simulink model "CF010A_GmTqArbn"  (R2013b)
settings: Solver=FixedStepDiscrete  SolverMode=SingleTasking  StartTime=0.0  StopTime=1  FixedStep=0.002  RelTol=1e-3
values from neighbouring files (symbols this model uses):
  ARCHGLBPRM_2MILLISEC_SEC_F32 = DataDict.Constant    [CF010A_GmTqArbn_DataDict.m]
  ESCCMDACTV_CNT_U08 = DataDict.Constant    [CF010A_GmTqArbn_DataDict.m]
  ESCCMDTMPLIMD_CNT_U08 = DataDict.Constant    [CF010A_GmTqArbn_DataDict.m]
  ESCTQCMDOVRLLIM_HWNWTMTR_F32 = DataDict.Constant    [CF010A_GmTqArbn_DataDict.m]
  FINALSLEWLWRLIM_HWNWTMTRPERSEC_F32 = DataDict.Constant    [CF010A_GmTqArbn_DataDict.m]
  GmTqArbnApaAssiScaEna = DataDict.Calibration    [CF010A_GmTqArbn_DataDict.m]
  GmTqArbnApaDampgScaEna = DataDict.Calibration    [CF010A_GmTqArbn_DataDict.m]
  GmTqArbnApaEnaRate = DataDict.Calibration    [CF010A_GmTqArbn_DataDict.m]
  GmTqArbnApaRtnScaEna = DataDict.Calibration    [CF010A_GmTqArbn_DataDict.m]
  GmTqArbnEscMaxTq = DataDict.Calibration    [CF010A_GmTqArbn_DataDict.m]
  GmTqArbnLkaSlewEna = DataDict.Calibration    [CF010A_GmTqArbn_DataDict.m]
  HWTQCMDOVRLLIM_HWNWTMTR_F32 = DataDict.Constant    [CF010A_GmTqArbn_DataDict.m]
  LKACMDHILIM_HWNWTMTR_F32 = DataDict.Constant    [CF010A_GmTqArbn_DataDict.m]
  LKASTACTV_CNT_U08 = DataDict.Constant    [CF010A_GmTqArbn_DataDict.m]
  LKATQCMDOVRLLIM_HWNWTMTR_F32 = DataDict.Constant    [CF010A_GmTqArbn_DataDict.m]
  MOTTQCMDOVRLLIM_MOTNWTMTR_F32 = DataDict.Constant    [CF010A_GmTqArbn_DataDict.m]
  OUTPCMDHILIM_ULS_F32 = DataDict.Constant    [CF010A_GmTqArbn_DataDict.m]
  OUTPCMDLOWRLIM_ULS_F32 = DataDict.Constant    [CF010A_GmTqArbn_DataDict.m]
  POSNSERVOSMOOTHMINLWRLIM_ULSPERSEC_F32 = DataDict.Constant    [CF010A_GmTqArbn_DataDict.m]
  VELDPTTQOVRLMTRCOFFS_HWNWTMTRPERSEC_F32 = DataDict.Constant    [CF010A_GmTqArbn_DataDict.m]
  VELDPTTQOVRLMTRCTQPERVEHSPD_HWNWTMTRPERSECPERKPH_F32 = DataDict.Constant    [CF010A_GmTqArbn_DataDict.m]
libraries: NxtrLim x11, NexteerUtilities x8, FixdToFloat x3, Fil x2, NxtrAbslt x2, simulink x2
(part 2 of 4)

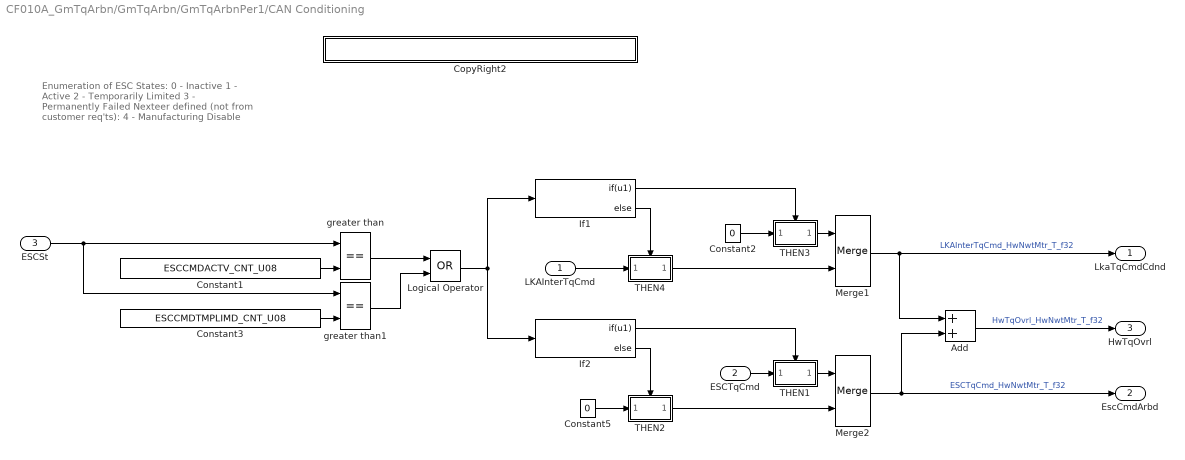
== system CF010A_GmTqArbn/GmTqArbn/GmTqArbnPer1/CAN Conditioning ==
  note: Enumeration of ESC States:
      |     0 - Inactive
      |     1 - Active
      |     2 - Temporarily Limited
      |     3 - Permanently Failed
      |
      | Nexteer defined (not from customer req'ts):
      |     4 - Manufacturing Disable
  LKAInterTqCmd : Inport
  ESCTqCmd : Inport  Port=2
  ESCSt : Inport  Port=3
  Add : Sum
  Constant1 : Constant  Value=ESCCMDACTV_CNT_U08
  Constant2 : Constant  Value=0  OutDataTypeStr=single
  Constant3 : Constant  Value=ESCCMDTMPLIMD_CNT_U08
  Constant5 : Constant  Value=0  OutDataTypeStr=single
  CopyRight2 : Subsystem  Description=|  mask(Copyright Information){none=on}
      | Copyright info block.                                               
      |                                                                     
      | Place copyright information at the top of every subsystem in design.
      mask prompts: none "No parameters"
      mask help: Place copyright information at the top of every subsystem in design.
      mask Display:
      | NxtrConf = 'Nexteer Confidential';
      | 
      | sys = bdroot; %handle for the current model ("system")
      | first = get_param(sys,'Created');
      | first = first(end-3:end);  %year is last four digits
      | 
      | last = get_param(sys,'LastModifiedDate');
      | if isempty(last)
      |     last = datestr(now,'yyyy');
      | else
      |     last = last(end-3:end);
      | end
      | 
      | if strcmp(first,last)
      |     fprintf('%s -- Copyright %s Nexteer',NxtrConf,first)
      | else
      |     fprintf('%s -- %s%s- %s Nexteer',NxtrConf,char(169),first,last)
      | end
  If1 : If  IfExpression=u1
  If2 : If  IfExpression=u1
  Logical Operator : Logic  Operator=OR  AllPortsSameDT=off  OutDataTypeStr=boolean
  Merge1 : Merge
  Merge2 : Merge
  THEN1 : Subsystem  RequirementInfo={} %GIDa_df789066_5626_4b2f_a61b_8784029d3cc8  TreatAsAtomicUnit=on  mask(pass thru, version Nov 30, 2012){nIn=1}
      mask prompts: nIn "Number of input signals"
      mask help:
      | This block passes its input straight through without modification.
      |
      | Enter the number of signals to pass through (integer 1 to 5).
      mask Callback nIn:
      | thisBlock = gcb;
      | a = get_param(thisBlock,'MaskValues');
      | b = cell2mat(a);
      | c = str2num(b);
      | 
      | if c<1 c=1; end
      | if c>5 c=5; end
      | 
      | for idx=1:c
      |     sIdx = num2str(idx);
      |     oldblock = [thisBlock '/In' sIdx];
      |     if strcmp(get_param(oldblock,'BlockType'),'Ground')
      |          newblock = 'built-in/Inport';
      |         pos = get_param(oldblock,'Position');
      |         orient = get_param(oldblock,'Orientation');
      |         delete_block(oldblock);
      |         add_block(newblock,oldblock,'Position',pos, 'Orientation',orient);
      |     end
      | 
      |     oldblock = [thisBlock '/Out' sIdx];
      |     if strcmp(get_param(oldblock,'BlockType'),'Terminator')
      |         newblock = 'built-in/Outport';
      |         pos = get_param(oldblock,'Position');
      |         orient = get_param(oldblock,'Orientation');
      |         delete_block(oldblock);
      |         add_block(newblock,oldblock,'Position',pos, 'Orientation',orient);
      |     end
      | end
      | 
      | for idx=c+1:5
      |     sIdx = num2str(idx);
      |     oldblock = [thisBlock '/In' sIdx];
      |     if strcmp(get_param(oldblock,'BlockType'),'Inport')
      |         newblock = 'built-in/Ground';
      |         pos = get_param(oldblock,'Position');
      |         orient = get_param(oldblock,'Orientation');
      |         delete_block(oldblock);
      |         add_block(newblock,oldblock,'Position',pos, 'Orientation',orient);
      |     end
      | 
      |     oldblock = [thisBlock '/Out' sIdx];
      |     if strcmp(get_param(oldblock,'BlockType'),'Outport')
      |         newblock = 'built-in/Terminator';
      |         pos = get_param(oldblock,'Position');
      |         orient = get_param(oldblock,'Orientation');
      |         delete_block(oldblock);
      |         add_block(newblock,oldblock,'Position',pos, 'Orientation',orient);
      |     end
      | end
      | 
      | 
      | 
      | clear thisBlock oldblock newblock orient pos a b c idx sIdx ;
      mask Display: fprintf('pass\nthru')
  THEN2 : Subsystem  RequirementInfo={} %GIDa_50ca75fe_c393_440b_9fca_2138a66effba  TreatAsAtomicUnit=on  mask(pass thru, version Nov 30, 2012){nIn=1}
      mask prompts: nIn "Number of input signals"
      mask help:
      | This block passes its input straight through without modification.
      |
      | Enter the number of signals to pass through (integer 1 to 5).
      mask Callback nIn:
      | thisBlock = gcb;
      | a = get_param(thisBlock,'MaskValues');
      | b = cell2mat(a);
      | c = str2num(b);
      | 
      | if c<1 c=1; end
      | if c>5 c=5; end
      | 
      | for idx=1:c
      |     sIdx = num2str(idx);
      |     oldblock = [thisBlock '/In' sIdx];
      |     if strcmp(get_param(oldblock,'BlockType'),'Ground')
      |          newblock = 'built-in/Inport';
      |         pos = get_param(oldblock,'Position');
      |         orient = get_param(oldblock,'Orientation');
      |         delete_block(oldblock);
      |         add_block(newblock,oldblock,'Position',pos, 'Orientation',orient);
      |     end
      | 
      |     oldblock = [thisBlock '/Out' sIdx];
      |     if strcmp(get_param(oldblock,'BlockType'),'Terminator')
      |         newblock = 'built-in/Outport';
      |         pos = get_param(oldblock,'Position');
      |         orient = get_param(oldblock,'Orientation');
      |         delete_block(oldblock);
      |         add_block(newblock,oldblock,'Position',pos, 'Orientation',orient);
      |     end
      | end
      | 
      | for idx=c+1:5
      |     sIdx = num2str(idx);
      |     oldblock = [thisBlock '/In' sIdx];
      |     if strcmp(get_param(oldblock,'BlockType'),'Inport')
      |         newblock = 'built-in/Ground';
      |         pos = get_param(oldblock,'Position');
      |         orient = get_param(oldblock,'Orientation');
      |         delete_block(oldblock);
      |         add_block(newblock,oldblock,'Position',pos, 'Orientation',orient);
      |     end
      | 
      |     oldblock = [thisBlock '/Out' sIdx];
      |     if strcmp(get_param(oldblock,'BlockType'),'Outport')
      |         newblock = 'built-in/Terminator';
      |         pos = get_param(oldblock,'Position');
      |         orient = get_param(oldblock,'Orientation');
      |         delete_block(oldblock);
      |         add_block(newblock,oldblock,'Position',pos, 'Orientation',orient);
      |     end
      | end
      | 
      | 
      | 
      | clear thisBlock oldblock newblock orient pos a b c idx sIdx ;
      mask Display: fprintf('pass\nthru')
  THEN3 : Subsystem  RequirementInfo={} %GIDa_81dcbbe4_bcf9_4683_b7ed_1b758c0b3447  TreatAsAtomicUnit=on  mask(pass thru, version Nov 30, 2012){nIn=1}
      mask prompts: nIn "Number of input signals"
      mask help:
      | This block passes its input straight through without modification.
      |
      | Enter the number of signals to pass through (integer 1 to 5).
      mask Callback nIn:
      | thisBlock = gcb;
      | a = get_param(thisBlock,'MaskValues');
      | b = cell2mat(a);
      | c = str2num(b);
      | 
      | if c<1 c=1; end
      | if c>5 c=5; end
      | 
      | for idx=1:c
      |     sIdx = num2str(idx);
      |     oldblock = [thisBlock '/In' sIdx];
      |     if strcmp(get_param(oldblock,'BlockType'),'Ground')
      |          newblock = 'built-in/Inport';
      |         pos = get_param(oldblock,'Position');
      |         orient = get_param(oldblock,'Orientation');
      |         delete_block(oldblock);
      |         add_block(newblock,oldblock,'Position',pos, 'Orientation',orient);
      |     end
      | 
      |     oldblock = [thisBlock '/Out' sIdx];
      |     if strcmp(get_param(oldblock,'BlockType'),'Terminator')
      |         newblock = 'built-in/Outport';
      |         pos = get_param(oldblock,'Position');
      |         orient = get_param(oldblock,'Orientation');
      |         delete_block(oldblock);
      |         add_block(newblock,oldblock,'Position',pos, 'Orientation',orient);
      |     end
      | end
      | 
      | for idx=c+1:5
      |     sIdx = num2str(idx);
      |     oldblock = [thisBlock '/In' sIdx];
      |     if strcmp(get_param(oldblock,'BlockType'),'Inport')
      |         newblock = 'built-in/Ground';
      |         pos = get_param(oldblock,'Position');
      |         orient = get_param(oldblock,'Orientation');
      |         delete_block(oldblock);
      |         add_block(newblock,oldblock,'Position',pos, 'Orientation',orient);
      |     end
      | 
      |     oldblock = [thisBlock '/Out' sIdx];
      |     if strcmp(get_param(oldblock,'BlockType'),'Outport')
      |         newblock = 'built-in/Terminator';
      |         pos = get_param(oldblock,'Position');
      |         orient = get_param(oldblock,'Orientation');
      |         delete_block(oldblock);
      |         add_block(newblock,oldblock,'Position',pos, 'Orientation',orient);
      |     end
      | end
      | 
      | 
      | 
      | clear thisBlock oldblock newblock orient pos a b c idx sIdx ;
      mask Display: fprintf('pass\nthru')
  THEN4 : Subsystem  RequirementInfo={} %GIDa_7b8aef20_5d37_42b0_b34b_35905273f895  TreatAsAtomicUnit=on  mask(pass thru, version Nov 30, 2012){nIn=1}
      mask prompts: nIn "Number of input signals"
      mask help:
      | This block passes its input straight through without modification.
      |
      | Enter the number of signals to pass through (integer 1 to 5).
      mask Callback nIn:
      | thisBlock = gcb;
      | a = get_param(thisBlock,'MaskValues');
      | b = cell2mat(a);
      | c = str2num(b);
      | 
      | if c<1 c=1; end
      | if c>5 c=5; end
      | 
      | for idx=1:c
      |     sIdx = num2str(idx);
      |     oldblock = [thisBlock '/In' sIdx];
      |     if strcmp(get_param(oldblock,'BlockType'),'Ground')
      |          newblock = 'built-in/Inport';
      |         pos = get_param(oldblock,'Position');
      |         orient = get_param(oldblock,'Orientation');
      |         delete_block(oldblock);
      |         add_block(newblock,oldblock,'Position',pos, 'Orientation',orient);
      |     end
      | 
      |     oldblock = [thisBlock '/Out' sIdx];
      |     if strcmp(get_param(oldblock,'BlockType'),'Terminator')
      |         newblock = 'built-in/Outport';
      |         pos = get_param(oldblock,'Position');
      |         orient = get_param(oldblock,'Orientation');
      |         delete_block(oldblock);
      |         add_block(newblock,oldblock,'Position',pos, 'Orientation',orient);
      |     end
      | end
      | 
      | for idx=c+1:5
      |     sIdx = num2str(idx);
      |     oldblock = [thisBlock '/In' sIdx];
      |     if strcmp(get_param(oldblock,'BlockType'),'Inport')
      |         newblock = 'built-in/Ground';
      |         pos = get_param(oldblock,'Position');
      |         orient = get_param(oldblock,'Orientation');
      |         delete_block(oldblock);
      |         add_block(newblock,oldblock,'Position',pos, 'Orientation',orient);
      |     end
      | 
      |     oldblock = [thisBlock '/Out' sIdx];
      |     if strcmp(get_param(oldblock,'BlockType'),'Outport')
      |         newblock = 'built-in/Terminator';
      |         pos = get_param(oldblock,'Position');
      |         orient = get_param(oldblock,'Orientation');
      |         delete_block(oldblock);
      |         add_block(newblock,oldblock,'Position',pos, 'Orientation',orient);
      |     end
      | end
      | 
      | 
      | 
      | clear thisBlock oldblock newblock orient pos a b c idx sIdx ;
      mask Display: fprintf('pass\nthru')
  greater than : RelationalOperator  Operator===  OutDataTypeStr=boolean
  greater than1 : RelationalOperator  Operator===  OutDataTypeStr=boolean
  LkaTqCmdCdnd : Outport
  EscCmdArbd : Outport  Port=2
  HwTqOvrl : Outport  Port=3
  wires:
  ESCSt/1 -> greater than/1, greater than1/1
  greater than/1 -> Logical Operator/1
  greater than1/1 -> Logical Operator/2
  THEN3/1(Out1) -> Merge1/1
  Constant2/1 -> THEN3/1(In1)
  If1/1 -> THEN3/Action
  LKAInterTqCmd/1 -> THEN4/1(In1)
  If1/2 -> THEN4/Action
  THEN4/1(Out1) -> Merge1/2
  Constant1/1 -> greater than/2
  Constant3/1 -> greater than1/2
  Logical Operator/1 -> If2/1, If1/1
  THEN1/1(Out1) -> Merge2/1
  If2/1 -> THEN1/Action
  If2/2 -> THEN2/Action
  THEN2/1(Out1) -> Merge2/2
  Merge2/1 -> Add/2, EscCmdArbd/1  "ESCTqCmd_HwNwtMtr_T_f32"
  Merge1/1 -> Add/1, LkaTqCmdCdnd/1  "LKAInterTqCmd_HwNwtMtr_T_f32"
  Add/1 -> HwTqOvrl/1  "HwTqOvrl_HwNwtMtr_T_f32"
  ESCTqCmd/1 -> THEN1/1(In1)
  Constant5/1 -> THEN2/1(In1)

== system CF010A_GmTqArbn/GmTqArbn/GmTqArbnPer1/CopyRight2 ==

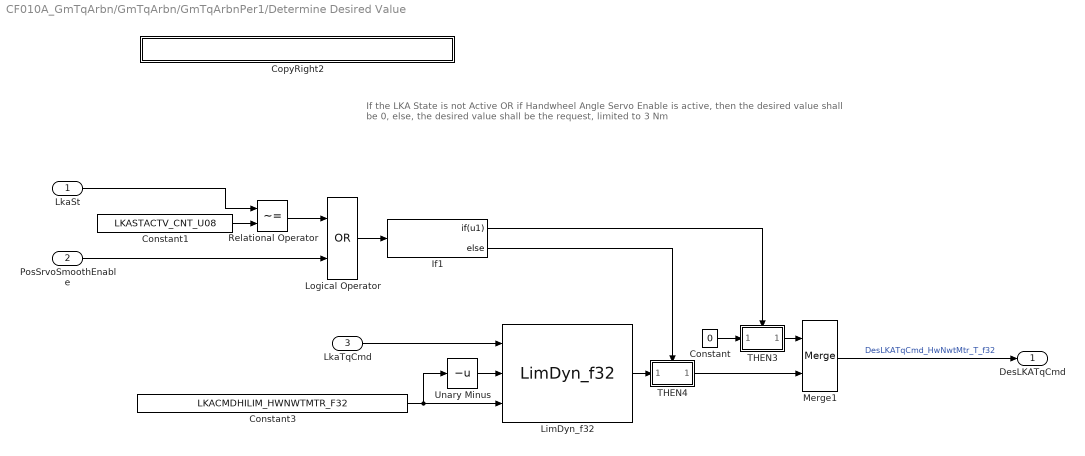
== system CF010A_GmTqArbn/GmTqArbn/GmTqArbnPer1/Determine Desired Value ==
  note: If the LKA State is not Active OR if Handwheel Angle Servo Enable is active, then the desired value shall be 0,
      | else, the desired value shall be the request, limited to 3 Nm
  LkaSt : Inport
  PosSrvoSmoothEnable : Inport  Port=2
  LkaTqCmd : Inport  Port=3
  Constant : Constant  Value=0  OutDataTypeStr=single
  Constant1 : Constant  Value=LKASTACTV_CNT_U08
  Constant3 : Constant  Value=LKACMDHILIM_HWNWTMTR_F32
  CopyRight2 : Subsystem  Description=|  mask(Copyright Information){none=on}
      | Copyright info block.                                               
      |                                                                     
      | Place copyright information at the top of every subsystem in design.
      mask prompts: none "No parameters"
      mask help: Place copyright information at the top of every subsystem in design.
      mask Display:
      | NxtrConf = 'Nexteer Confidential';
      | 
      | sys = bdroot; %handle for the current model ("system")
      | first = get_param(sys,'Created');
      | first = first(end-3:end);  %year is last four digits
      | 
      | last = get_param(sys,'LastModifiedDate');
      | if isempty(last)
      |     last = datestr(now,'yyyy');
      | else
      |     last = last(end-3:end);
      | end
      | 
      | if strcmp(first,last)
      |     fprintf('%s -- Copyright %s Nexteer',NxtrConf,first)
      | else
      |     fprintf('%s -- %s%s- %s Nexteer',NxtrConf,char(169),first,last)
      | end
  If1 : If  IfExpression=u1
  LimDyn_f32 : NxtrLim/LimDyn_f32
  Logical Operator : Logic  Operator=OR  AllPortsSameDT=off  OutDataTypeStr=boolean
  Merge1 : Merge
  Relational Operator : RelationalOperator  Operator=~=  OutDataTypeStr=boolean
  THEN3 : Subsystem  RequirementInfo={} %GIDa_0606f6db_8c1b_4172_ad9d_e86aee79a80c  TreatAsAtomicUnit=on  mask(pass thru, version Nov 30, 2012){nIn=1}
      mask prompts: nIn "Number of input signals"
      mask help:
      | This block passes its input straight through without modification.
      |
      | Enter the number of signals to pass through (integer 1 to 5).
      mask Callback nIn:
      | thisBlock = gcb;
      | a = get_param(thisBlock,'MaskValues');
      | b = cell2mat(a);
      | c = str2num(b);
      | 
      | if c<1 c=1; end
      | if c>5 c=5; end
      | 
      | for idx=1:c
      |     sIdx = num2str(idx);
      |     oldblock = [thisBlock '/In' sIdx];
      |     if strcmp(get_param(oldblock,'BlockType'),'Ground')
      |          newblock = 'built-in/Inport';
      |         pos = get_param(oldblock,'Position');
      |         orient = get_param(oldblock,'Orientation');
      |         delete_block(oldblock);
      |         add_block(newblock,oldblock,'Position',pos, 'Orientation',orient);
      |     end
      | 
      |     oldblock = [thisBlock '/Out' sIdx];
      |     if strcmp(get_param(oldblock,'BlockType'),'Terminator')
      |         newblock = 'built-in/Outport';
      |         pos = get_param(oldblock,'Position');
      |         orient = get_param(oldblock,'Orientation');
      |         delete_block(oldblock);
      |         add_block(newblock,oldblock,'Position',pos, 'Orientation',orient);
      |     end
      | end
      | 
      | for idx=c+1:5
      |     sIdx = num2str(idx);
      |     oldblock = [thisBlock '/In' sIdx];
      |     if strcmp(get_param(oldblock,'BlockType'),'Inport')
      |         newblock = 'built-in/Ground';
      |         pos = get_param(oldblock,'Position');
      |         orient = get_param(oldblock,'Orientation');
      |         delete_block(oldblock);
      |         add_block(newblock,oldblock,'Position',pos, 'Orientation',orient);
      |     end
      | 
      |     oldblock = [thisBlock '/Out' sIdx];
      |     if strcmp(get_param(oldblock,'BlockType'),'Outport')
      |         newblock = 'built-in/Terminator';
      |         pos = get_param(oldblock,'Position');
      |         orient = get_param(oldblock,'Orientation');
      |         delete_block(oldblock);
      |         add_block(newblock,oldblock,'Position',pos, 'Orientation',orient);
      |     end
      | end
      | 
      | 
      | 
      | clear thisBlock oldblock newblock orient pos a b c idx sIdx ;
      mask Display: fprintf('pass\nthru')
  THEN4 : Subsystem  RequirementInfo={} %GIDa_83d48c39_410e_4c17_a4dc_2ab1cb247f6f  TreatAsAtomicUnit=on  mask(pass thru, version Nov 30, 2012){nIn=1}
      mask prompts: nIn "Number of input signals"
      mask help:
      | This block passes its input straight through without modification.
      |
      | Enter the number of signals to pass through (integer 1 to 5).
      mask Callback nIn:
      | thisBlock = gcb;
      | a = get_param(thisBlock,'MaskValues');
      | b = cell2mat(a);
      | c = str2num(b);
      | 
      | if c<1 c=1; end
      | if c>5 c=5; end
      | 
      | for idx=1:c
      |     sIdx = num2str(idx);
      |     oldblock = [thisBlock '/In' sIdx];
      |     if strcmp(get_param(oldblock,'BlockType'),'Ground')
      |          newblock = 'built-in/Inport';
      |         pos = get_param(oldblock,'Position');
      |         orient = get_param(oldblock,'Orientation');
      |         delete_block(oldblock);
      |         add_block(newblock,oldblock,'Position',pos, 'Orientation',orient);
      |     end
      | 
      |     oldblock = [thisBlock '/Out' sIdx];
      |     if strcmp(get_param(oldblock,'BlockType'),'Terminator')
      |         newblock = 'built-in/Outport';
      |         pos = get_param(oldblock,'Position');
      |         orient = get_param(oldblock,'Orientation');
      |         delete_block(oldblock);
      |         add_block(newblock,oldblock,'Position',pos, 'Orientation',orient);
      |     end
      | end
      | 
      | for idx=c+1:5
      |     sIdx = num2str(idx);
      |     oldblock = [thisBlock '/In' sIdx];
      |     if strcmp(get_param(oldblock,'BlockType'),'Inport')
      |         newblock = 'built-in/Ground';
      |         pos = get_param(oldblock,'Position');
      |         orient = get_param(oldblock,'Orientation');
      |         delete_block(oldblock);
      |         add_block(newblock,oldblock,'Position',pos, 'Orientation',orient);
      |     end
      | 
      |     oldblock = [thisBlock '/Out' sIdx];
      |     if strcmp(get_param(oldblock,'BlockType'),'Outport')
      |         newblock = 'built-in/Terminator';
      |         pos = get_param(oldblock,'Position');
      |         orient = get_param(oldblock,'Orientation');
      |         delete_block(oldblock);
      |         add_block(newblock,oldblock,'Position',pos, 'Orientation',orient);
      |     end
      | end
      | 
      | 
      | 
      | clear thisBlock oldblock newblock orient pos a b c idx sIdx ;
      mask Display: fprintf('pass\nthru')
  Unary Minus : UnaryMinus
  DesLKATqCmd : Outport
  wires:
  PosSrvoSmoothEnable/1 -> Logical Operator/2
  Relational Operator/1 -> Logical Operator/1
  Logical Operator/1 -> If1/1
  Merge1/1 -> DesLKATqCmd/1  "DesLKATqCmd_HwNwtMtr_T_f32"
  LkaTqCmd/1 -> LimDyn_f32/1
  LkaSt/1 -> Relational Operator/1
  Constant1/1 -> Relational Operator/2
  THEN3/1(Out1) -> Merge1/1
  Constant/1 -> THEN3/1(In1)
  If1/1 -> THEN3/Action
  LimDyn_f32/1 -> THEN4/1(In1)
  If1/2 -> THEN4/Action
  THEN4/1(Out1) -> Merge1/2
  Constant3/1 -> Unary Minus/1, LimDyn_f32/3
  Unary Minus/1 -> LimDyn_f32/2

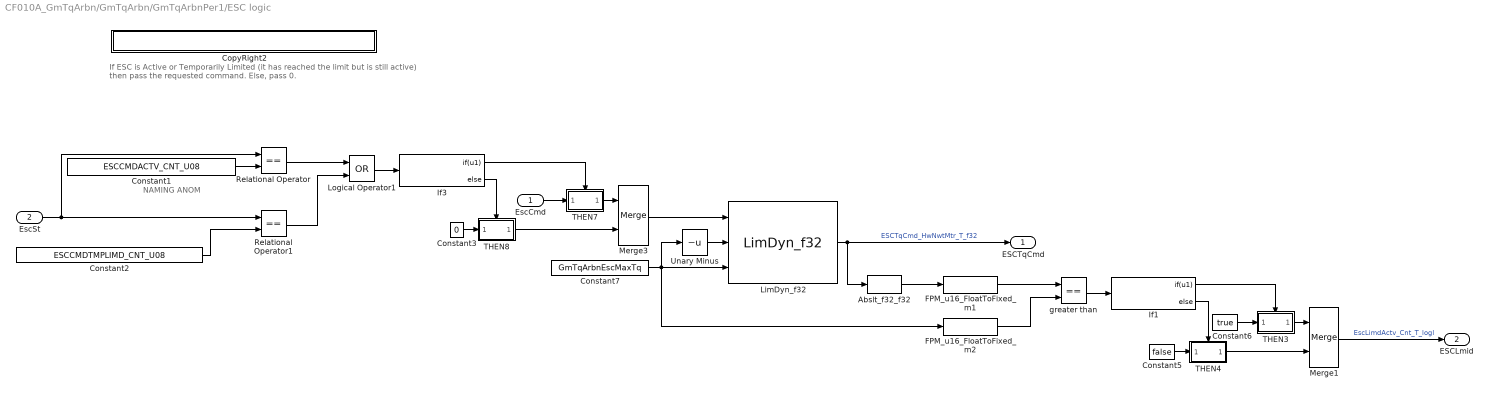
== system CF010A_GmTqArbn/GmTqArbn/GmTqArbnPer1/ESC logic ==
  note: NAMING ANOM
  note: If ESC is Active or Temporarily Limited (it has reached the limit but is still active)
      |   then pass the requested command.
      | Else,
      |   pass 0.
  EscCmd : Inport
  EscSt : Inport  Port=2
  Abslt_f32_f32 : NxtrAbslt/Abslt_f32_f32  SFunctionSpec=single y1 = Abslt_f32_f32(single u1)
      settings: AttributesFormatString=%<Name>
  Constant1 : Constant  Value=ESCCMDACTV_CNT_U08
  Constant2 : Constant  Value=ESCCMDTMPLIMD_CNT_U08
  Constant3 : Constant  Value=0  OutDataTypeStr=single
  Constant5 : Constant  Value=false  OutDataTypeStr=boolean
  Constant6 : Constant  Value=true  OutDataTypeStr=boolean
  Constant7 : Constant  Value=GmTqArbnEscMaxTq
  CopyRight2 : Subsystem  Description=|  mask(Copyright Information){none=on}
      | Copyright info block.                                               
      |                                                                     
      | Place copyright information at the top of every subsystem in design.
      mask prompts: none "No parameters"
      mask help: Place copyright information at the top of every subsystem in design.
      mask Display:
      | NxtrConf = 'Nexteer Confidential';
      | 
      | sys = bdroot; %handle for the current model ("system")
      | first = get_param(sys,'Created');
      | first = first(end-3:end);  %year is last four digits
      | 
      | last = get_param(sys,'LastModifiedDate');
      | if isempty(last)
      |     last = datestr(now,'yyyy');
      | else
      |     last = last(end-3:end);
      | end
      | 
      | if strcmp(first,last)
      |     fprintf('%s -- Copyright %s Nexteer',NxtrConf,first)
      | else
      |     fprintf('%s -- %s%s- %s Nexteer',NxtrConf,char(169),first,last)
      | end
  FPM_u16_FloatToFixed_m1 : NexteerUtilities/Fixed Point Math Conversions/FPM_u16_FloatToFixed_m  SFunctionSpec=uint16 y1 = FPM_u16_FloatToFixed_m(single u1, single p1)  Param1=13
      settings: AttributesFormatString=u16_FloatToFixed
  FPM_u16_FloatToFixed_m2 : NexteerUtilities/Fixed Point Math Conversions/FPM_u16_FloatToFixed_m  SFunctionSpec=uint16 y1 = FPM_u16_FloatToFixed_m(single u1, single p1)  Param1=13
      settings: AttributesFormatString=u16_FloatToFixed
  If1 : If  IfExpression=u1
  If3 : If  IfExpression=u1
  LimDyn_f32 : NxtrLim/LimDyn_f32
  Logical Operator1 : Logic  Operator=OR  AllPortsSameDT=off  OutDataTypeStr=boolean
  Merge1 : Merge
  Merge3 : Merge
  Relational Operator : RelationalOperator  Operator===  OutDataTypeStr=boolean
  Relational Operator1 : RelationalOperator  Operator===  OutDataTypeStr=boolean
  THEN3 : Subsystem  RequirementInfo={} %GIDa_7cb0b7aa_377c_45b6_abd8_3cab6ad4e216  TreatAsAtomicUnit=on  mask(pass thru, version Nov 30, 2012){nIn=1}
      mask prompts: nIn "Number of input signals"
      mask help:
      | This block passes its input straight through without modification.
      |
      | Enter the number of signals to pass through (integer 1 to 5).
      mask Callback nIn:
      | thisBlock = gcb;
      | a = get_param(thisBlock,'MaskValues');
      | b = cell2mat(a);
      | c = str2num(b);
      | 
      | if c<1 c=1; end
      | if c>5 c=5; end
      | 
      | for idx=1:c
      |     sIdx = num2str(idx);
      |     oldblock = [thisBlock '/In' sIdx];
      |     if strcmp(get_param(oldblock,'BlockType'),'Ground')
      |          newblock = 'built-in/Inport';
      |         pos = get_param(oldblock,'Position');
      |         orient = get_param(oldblock,'Orientation');
      |         delete_block(oldblock);
      |         add_block(newblock,oldblock,'Position',pos, 'Orientation',orient);
      |     end
      | 
      |     oldblock = [thisBlock '/Out' sIdx];
      |     if strcmp(get_param(oldblock,'BlockType'),'Terminator')
      |         newblock = 'built-in/Outport';
      |         pos = get_param(oldblock,'Position');
      |         orient = get_param(oldblock,'Orientation');
      |         delete_block(oldblock);
      |         add_block(newblock,oldblock,'Position',pos, 'Orientation',orient);
      |     end
      | end
      | 
      | for idx=c+1:5
      |     sIdx = num2str(idx);
      |     oldblock = [thisBlock '/In' sIdx];
      |     if strcmp(get_param(oldblock,'BlockType'),'Inport')
      |         newblock = 'built-in/Ground';
      |         pos = get_param(oldblock,'Position');
      |         orient = get_param(oldblock,'Orientation');
      |         delete_block(oldblock);
      |         add_block(newblock,oldblock,'Position',pos, 'Orientation',orient);
      |     end
      | 
      |     oldblock = [thisBlock '/Out' sIdx];
      |     if strcmp(get_param(oldblock,'BlockType'),'Outport')
      |         newblock = 'built-in/Terminator';
      |         pos = get_param(oldblock,'Position');
      |         orient = get_param(oldblock,'Orientation');
      |         delete_block(oldblock);
      |         add_block(newblock,oldblock,'Position',pos, 'Orientation',orient);
      |     end
      | end
      | 
      | 
      | 
      | clear thisBlock oldblock newblock orient pos a b c idx sIdx ;
      mask Display: fprintf('pass\nthru')
  THEN4 : Subsystem  RequirementInfo={} %GIDa_ec69e255_cda7_4831_824b_afe7668fc332  TreatAsAtomicUnit=on  mask(pass thru, version Nov 30, 2012){nIn=1}
      mask prompts: nIn "Number of input signals"
      mask help:
      | This block passes its input straight through without modification.
      |
      | Enter the number of signals to pass through (integer 1 to 5).
      mask Callback nIn:
      | thisBlock = gcb;
      | a = get_param(thisBlock,'MaskValues');
      | b = cell2mat(a);
      | c = str2num(b);
      | 
      | if c<1 c=1; end
      | if c>5 c=5; end
      | 
      | for idx=1:c
      |     sIdx = num2str(idx);
      |     oldblock = [thisBlock '/In' sIdx];
      |     if strcmp(get_param(oldblock,'BlockType'),'Ground')
      |          newblock = 'built-in/Inport';
      |         pos = get_param(oldblock,'Position');
      |         orient = get_param(oldblock,'Orientation');
      |         delete_block(oldblock);
      |         add_block(newblock,oldblock,'Position',pos, 'Orientation',orient);
      |     end
      | 
      |     oldblock = [thisBlock '/Out' sIdx];
      |     if strcmp(get_param(oldblock,'BlockType'),'Terminator')
      |         newblock = 'built-in/Outport';
      |         pos = get_param(oldblock,'Position');
      |         orient = get_param(oldblock,'Orientation');
      |         delete_block(oldblock);
      |         add_block(newblock,oldblock,'Position',pos, 'Orientation',orient);
      |     end
      | end
      | 
      | for idx=c+1:5
      |     sIdx = num2str(idx);
      |     oldblock = [thisBlock '/In' sIdx];
      |     if strcmp(get_param(oldblock,'BlockType'),'Inport')
      |         newblock = 'built-in/Ground';
      |         pos = get_param(oldblock,'Position');
      |         orient = get_param(oldblock,'Orientation');
      |         delete_block(oldblock);
      |         add_block(newblock,oldblock,'Position',pos, 'Orientation',orient);
      |     end
      | 
      |     oldblock = [thisBlock '/Out' sIdx];
      |     if strcmp(get_param(oldblock,'BlockType'),'Outport')
      |         newblock = 'built-in/Terminator';
      |         pos = get_param(oldblock,'Position');
      |         orient = get_param(oldblock,'Orientation');
      |         delete_block(oldblock);
      |         add_block(newblock,oldblock,'Position',pos, 'Orientation',orient);
      |     end
      | end
      | 
      | 
      | 
      | clear thisBlock oldblock newblock orient pos a b c idx sIdx ;
      mask Display: fprintf('pass\nthru')
  THEN7 : Subsystem  RequirementInfo={} %GIDa_df5e48f9_4d3d_4963_bded_9993ee7d5991  TreatAsAtomicUnit=on  mask(pass thru, version Nov 30, 2012){nIn=1}
      mask prompts: nIn "Number of input signals"
      mask help:
      | This block passes its input straight through without modification.
      |
      | Enter the number of signals to pass through (integer 1 to 5).
      mask Callback nIn:
      | thisBlock = gcb;
      | a = get_param(thisBlock,'MaskValues');
      | b = cell2mat(a);
      | c = str2num(b);
      | 
      | if c<1 c=1; end
      | if c>5 c=5; end
      | 
      | for idx=1:c
      |     sIdx = num2str(idx);
      |     oldblock = [thisBlock '/In' sIdx];
      |     if strcmp(get_param(oldblock,'BlockType'),'Ground')
      |          newblock = 'built-in/Inport';
      |         pos = get_param(oldblock,'Position');
      |         orient = get_param(oldblock,'Orientation');
      |         delete_block(oldblock);
      |         add_block(newblock,oldblock,'Position',pos, 'Orientation',orient);
      |     end
      | 
      |     oldblock = [thisBlock '/Out' sIdx];
      |     if strcmp(get_param(oldblock,'BlockType'),'Terminator')
      |         newblock = 'built-in/Outport';
      |         pos = get_param(oldblock,'Position');
      |         orient = get_param(oldblock,'Orientation');
      |         delete_block(oldblock);
      |         add_block(newblock,oldblock,'Position',pos, 'Orientation',orient);
      |     end
      | end
      | 
      | for idx=c+1:5
      |     sIdx = num2str(idx);
      |     oldblock = [thisBlock '/In' sIdx];
      |     if strcmp(get_param(oldblock,'BlockType'),'Inport')
      |         newblock = 'built-in/Ground';
      |         pos = get_param(oldblock,'Position');
      |         orient = get_param(oldblock,'Orientation');
      |         delete_block(oldblock);
      |         add_block(newblock,oldblock,'Position',pos, 'Orientation',orient);
      |     end
      | 
      |     oldblock = [thisBlock '/Out' sIdx];
      |     if strcmp(get_param(oldblock,'BlockType'),'Outport')
      |         newblock = 'built-in/Terminator';
      |         pos = get_param(oldblock,'Position');
      |         orient = get_param(oldblock,'Orientation');
      |         delete_block(oldblock);
      |         add_block(newblock,oldblock,'Position',pos, 'Orientation',orient);
      |     end
      | end
      | 
      | 
      | 
      | clear thisBlock oldblock newblock orient pos a b c idx sIdx ;
      mask Display: fprintf('pass\nthru')
  THEN8 : Subsystem  RequirementInfo={} %GIDa_058d061c_9a6a_4e56_a7df_5107ed3b1fbe  TreatAsAtomicUnit=on  mask(pass thru, version Nov 30, 2012){nIn=1}
      mask prompts: nIn "Number of input signals"
      mask help:
      | This block passes its input straight through without modification.
      |
      | Enter the number of signals to pass through (integer 1 to 5).
      mask Callback nIn:
      | thisBlock = gcb;
      | a = get_param(thisBlock,'MaskValues');
      | b = cell2mat(a);
      | c = str2num(b);
      | 
      | if c<1 c=1; end
      | if c>5 c=5; end
      | 
      | for idx=1:c
      |     sIdx = num2str(idx);
      |     oldblock = [thisBlock '/In' sIdx];
      |     if strcmp(get_param(oldblock,'BlockType'),'Ground')
      |          newblock = 'built-in/Inport';
      |         pos = get_param(oldblock,'Position');
      |         orient = get_param(oldblock,'Orientation');
      |         delete_block(oldblock);
      |         add_block(newblock,oldblock,'Position',pos, 'Orientation',orient);
      |     end
      | 
      |     oldblock = [thisBlock '/Out' sIdx];
      |     if strcmp(get_param(oldblock,'BlockType'),'Terminator')
      |         newblock = 'built-in/Outport';
      |         pos = get_param(oldblock,'Position');
      |         orient = get_param(oldblock,'Orientation');
      |         delete_block(oldblock);
      |         add_block(newblock,oldblock,'Position',pos, 'Orientation',orient);
      |     end
      | end
      | 
      | for idx=c+1:5
      |     sIdx = num2str(idx);
      |     oldblock = [thisBlock '/In' sIdx];
      |     if strcmp(get_param(oldblock,'BlockType'),'Inport')
      |         newblock = 'built-in/Ground';
      |         pos = get_param(oldblock,'Position');
      |         orient = get_param(oldblock,'Orientation');
      |         delete_block(oldblock);
      |         add_block(newblock,oldblock,'Position',pos, 'Orientation',orient);
      |     end
      | 
      |     oldblock = [thisBlock '/Out' sIdx];
      |     if strcmp(get_param(oldblock,'BlockType'),'Outport')
      |         newblock = 'built-in/Terminator';
      |         pos = get_param(oldblock,'Position');
      |         orient = get_param(oldblock,'Orientation');
      |         delete_block(oldblock);
      |         add_block(newblock,oldblock,'Position',pos, 'Orientation',orient);
      |     end
      | end
      | 
      | 
      | 
      | clear thisBlock oldblock newblock orient pos a b c idx sIdx ;
      mask Display: fprintf('pass\nthru')
  Unary Minus : UnaryMinus
  greater than : RelationalOperator  Operator===  OutDataTypeStr=boolean
  ESCTqCmd : Outport
  ESCLmid : Outport  Port=2
  wires:
  Abslt_f32_f32/1 -> FPM_u16_FloatToFixed_m1/1
  EscSt/1 -> Relational Operator1/1, Relational Operator/1
  Relational Operator/1 -> Logical Operator1/1
  Relational Operator1/1 -> Logical Operator1/2
  Logical Operator1/1 -> If3/1
  Merge1/1 -> ESCLmid/1  "EscLimdActv_Cnt_T_logl"
  LimDyn_f32/1 -> Abslt_f32_f32/1, ESCTqCmd/1  "ESCTqCmd_HwNwtMtr_T_f32"
  Constant1/1 -> Relational Operator/2
  Constant2/1 -> Relational Operator1/2
  THEN7/1(Out1) -> Merge3/1
  EscCmd/1 -> THEN7/1(In1)
  If3/1 -> THEN7/Action
  Constant3/1 -> THEN8/1(In1)
  If3/2 -> THEN8/Action
  THEN8/1(Out1) -> Merge3/2
  Constant7/1 -> FPM_u16_FloatToFixed_m2/1, Unary Minus/1, LimDyn_f32/3
  THEN3/1(Out1) -> Merge1/1
  Constant6/1 -> THEN3/1(In1)
  If1/1 -> THEN3/Action
  Constant5/1 -> THEN4/1(In1)
  If1/2 -> THEN4/Action
  THEN4/1(Out1) -> Merge1/2
  greater than/1 -> If1/1
  Merge3/1 -> LimDyn_f32/1
  Unary Minus/1 -> LimDyn_f32/2
  FPM_u16_FloatToFixed_m1/1 -> greater than/1
  FPM_u16_FloatToFixed_m2/1 -> greater than/2
